simulink model "SMCControllerEH"  (R2022b)
settings: Solver=ode14x  StartTime=0.0  StopTime=simulationTime  FixedStep=sampleTime  RelTol=1e-6  AbsTol=1e-9
values from neighbouring files (symbols this model uses):
  chi = 0.05    [Basinofattraction.m]    (also in MainCEoptCase2_FOSMC.m; MainCEoptCase2_SMC.m; MainGAoptCase2_FOSMC.m; MainGAoptCase2_SMC.m)
  dxdisp0 = 0.0    (= 0)    [MainCEoptCase2_FOSMC.m]    (also in MainCEoptCase2_SMC.m; MainGAoptCase2_FOSMC.m; MainGAoptCase2_SMC.m)
  f_ref = 0.2    [Basinofattraction.m]    (also in MainCEoptCase2_FOSMC.m; MainCEoptCase2_SMC.m; MainGAoptCase2_FOSMC.m; MainGAoptCase2_SMC.m)
  fa = 0.2    [Basinofattraction.m]    (also in MainCEoptCase2_FOSMC.m; MainCEoptCase2_SMC.m; MainGAoptCase2_FOSMC.m; MainGAoptCase2_SMC.m)
  k = Xopt(1)    [Basinofattraction.m]    (also in MainCEoptCase2_FOSMC.m = x(1); MainCEoptCase2_SMC.m = x(1); MainGAoptCase2_FOSMC.m = x(1); MainGAoptCase2_SMC.m = x(1))
  kappa = 0.5    [Basinofattraction.m]    (also in MainCEoptCase2_FOSMC.m; MainCEoptCase2_SMC.m; MainGAoptCase2_FOSMC.m; MainGAoptCase2_SMC.m)
  ksi = 0.01    [Basinofattraction.m]    (also in MainCEoptCase2_FOSMC.m; MainCEoptCase2_SMC.m; MainGAoptCase2_FOSMC.m; MainGAoptCase2_SMC.m)
  lambda = 0.05    [Basinofattraction.m]    (also in MainCEoptCase2_FOSMC.m; MainCEoptCase2_SMC.m; MainGAoptCase2_FOSMC.m; MainGAoptCase2_SMC.m)
  lambda1 = Xopt(2)    [Basinofattraction.m]    (also in MainCEoptCase2_FOSMC.m = x(2); MainCEoptCase2_SMC.m = x(2); MainGAoptCase2_FOSMC.m = x(2); MainGAoptCase2_SMC.m = x(2))
  Omega_ref = 0.8    [Basinofattraction.m]    (also in MainCEoptCase2_FOSMC.m; MainCEoptCase2_SMC.m; MainGAoptCase2_FOSMC.m; MainGAoptCase2_SMC.m)
  sampleTime = 0.1    [Basinofattraction.m]    (also in MainCEoptCase2_FOSMC.m; MainCEoptCase2_SMC.m; MainGAoptCase2_FOSMC.m; MainGAoptCase2_SMC.m)
  xdisp0 = 1.0    (= 1)    [MainCEoptCase2_FOSMC.m]    (also in MainCEoptCase2_SMC.m; MainGAoptCase2_FOSMC.m; MainGAoptCase2_SMC.m)
settings Model: Creator=julio  LastModifiedBy=Usuario
settings SolverCC: AutoScaleAbsTol=off  InitialStep=sampleTime  AlgebraicLoopSolver=TrustRegion
settings DataIOCC: ReturnWorkspaceOutputs=off
settings OptimizationCC: LifeSpan=inf
settings DebuggingCC: UnconnectedInputMsg=warning  UnconnectedOutputMsg=warning  UnconnectedLineMsg=warning  SFUnexpectedBacktrackingDiag=warning  SFNoUnconditionalDefaultTransitionDiag=warning  SFMachineParentedDataDiag=warning  ArithmeticOperatorsInVariantConditions=warning
settings ModelReferenceCC: EnableRefExpFcnMdlSchedulingChecks=on
settings SFSimCC: SimUseLocalCustomCode=off  CustomCodeUndefinedFunction=UseInterfaceOnly
settings RTWCC: RTWUseLocalCustomCode=off
settings CodeAppCC: StateflowObjectComments=on
settings GRTTargetCC: TargetLangStandard=C89/C90 (ANSI)
settings ConfigComp: CovMetricSettings=dw  CovSaveCumulativeToWorkspaceVar=on  CovSaveSingleToWorkspaceVar=on  CovExternalEMLEnable=off

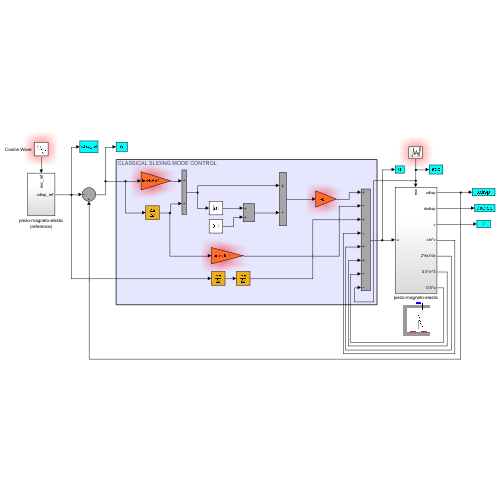
[thumbnail: Simulink's stored preview of the top-level diagram]
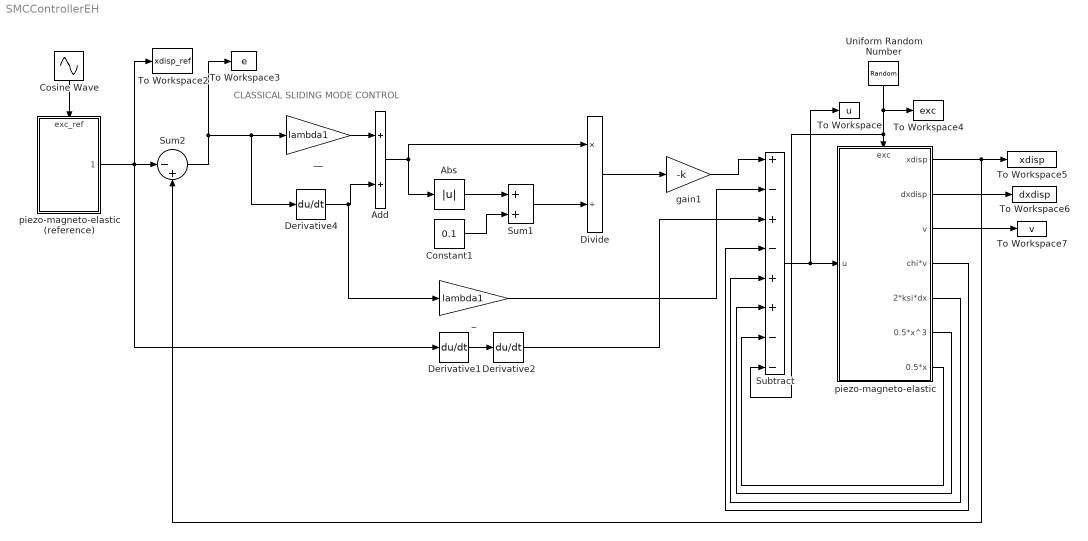
== system SMCControllerEH ==
  note: CLASSICAL SLIDING MODE CONTROL
  Abs : Abs  SaturateOnIntegerOverflow=off
  Add : Sum
  Constant1 : Constant  Value=0.1
  Cosine Wave : Sin  Amplitude=f_ref  Frequency=Omega_ref  SampleTime=0
  Derivative1 : Derivative
  Derivative2 : Derivative
  Derivative4 : Derivative
  Divide : Product  Inputs=*/
  Subtract : Sum  Inputs=+-+-++--
  Sum1 : Sum
  Sum2 : Sum  Inputs=|-+
  To Workspace : ToWorkspace  VariableName=u  SampleTime=-1
  To Workspace2 : ToWorkspace  VariableName=xdisp_ref  SampleTime=-1
  To Workspace3 : ToWorkspace  VariableName=e  SampleTime=-1
  To Workspace4 : ToWorkspace  VariableName=exc  SampleTime=-1
  To Workspace5 : ToWorkspace  VariableName=xdisp  SampleTime=-1
  To Workspace6 : ToWorkspace  VariableName=dxdisp  SampleTime=-1
  To Workspace7 : ToWorkspace  VariableName=v  SampleTime=-1
  Uniform Random Number : UniformRandomNumber  Minimum=-fa  Maximum=fa  Seed=1  SampleTime=sampleTime
  _ : Gain  Gain=lambda1
  __ : Gain  Gain=lambda1
  gain1 : Gain  Gain=-k
  piezo-magneto-elastic : Subsystem
      settings: PortSchema="{\"entries\":[{\"content\":{\"sides\":[{\"content\":{\"connectorIds\":[\"In1\"]},\"type\":\"ConnectorPlacement.EquallySpacedRectSide\",\"uuid\":\"c2ba6895-4fe1-43b2-9166-bfc98075714a\"},{\"content\":{\"connectorIds\":[\"Out1\",\"Out2\",\"Out3\",\"Out4\",\"Out5\",\"Out6\",\"Out7\"],\"side\":\"RIGHT\"},\"type\":\"ConnectorPlacement.EquallySpacedRectSide\",\"uuid\":\"f318010f-5345-4abb-8ec4-2c3ff83e3584\"},{\"content\":{\"connectorIds\":[\"In2\"],\"side\":\"TOP\"},\"type\":\"ConnectorPlacement.EquallySpacedRectSide\",\"uuid\":\"166745b2-692d-46bd-9a0d-c3d5b18ab8b7\"}]},\"type\":\"ConnectorPlacement.EquallySpacedConnector\",\"uuid\":\"a1a091f7-104a-4664-af8a-63d268c77923\"}],\"packageUris\":[\"http://schema.mathworks.com/mf0/Connector/R2020b\"],\"version\":\"1.0\"}"
  piezo-magneto-elastic (reference) : Subsystem
      settings: PortSchema="{\"entries\":[{\"content\":{\"sides\":[{\"content\":{\"connectorIds\":[]},\"type\":\"ConnectorPlacement.EquallySpacedRectSide\",\"uuid\":\"2fa27d44-66dd-459a-a915-b9e739ab4464\"},{\"content\":{\"connectorIds\":[\"Out1\"],\"side\":\"RIGHT\"},\"type\":\"ConnectorPlacement.EquallySpacedRectSide\",\"uuid\":\"143cbf88-99f3-4a4f-90c8-d8dcff3037ad\"},{\"content\":{\"connectorIds\":[\"In1\"],\"side\":\"TOP\"},\"type\":\"ConnectorPlacement.EquallySpacedRectSide\",\"uuid\":\"0f1da41b-b693-4442-9f27-75426a8f7a9a\"}]},\"type\":\"ConnectorPlacement.EquallySpacedConnector\",\"uuid\":\"82ec817d-257e-4c4b-88fa-5616da8b4759\"}],\"packageUris\":[\"http://schema.mathworks.com/mf0/Connector/R2020b\"],\"version\":\"1.0\"}"
  wires:
  Subtract/1 -> piezo-magneto-elastic/1(u), To Workspace/1
  __/1 -> Add/1
  Derivative4/1 -> _/1, Add/2
  gain1/1 -> Subtract/1
  Add/1 -> Divide/1, Abs/1
  Divide/1 -> gain1/1
  Abs/1 -> Sum1/1
  Sum1/1 -> Divide/2
  Constant1/1 -> Sum1/2
  Sum2/1 -> Derivative4/1, __/1, To Workspace3/1
  Derivative1/1 -> Derivative2/1
  Derivative2/1 -> Subtract/3
  _/1 -> Subtract/2
  piezo-magneto-elastic/4(chi*v) -> Subtract/4
  piezo-magneto-elastic/5(2*ksi*dx) -> Subtract/5
  piezo-magneto-elastic/6(0.5*x^3) -> Subtract/6
  piezo-magneto-elastic/7(0.5*x) -> Subtract/7
  piezo-magneto-elastic (reference)/1(xdisp_ref) -> To Workspace2/1, Sum2/1, Derivative1/1
  Cosine Wave/1 -> piezo-magneto-elastic (reference)/1(exc_ref)
  piezo-magneto-elastic/1(xdisp) -> Sum2/2, To Workspace5/1
  piezo-magneto-elastic/2(dxdisp) -> To Workspace6/1
  piezo-magneto-elastic/3(v) -> To Workspace7/1
  Uniform Random Number/1 -> Subtract/8, piezo-magneto-elastic/2(exc), To Workspace4/1

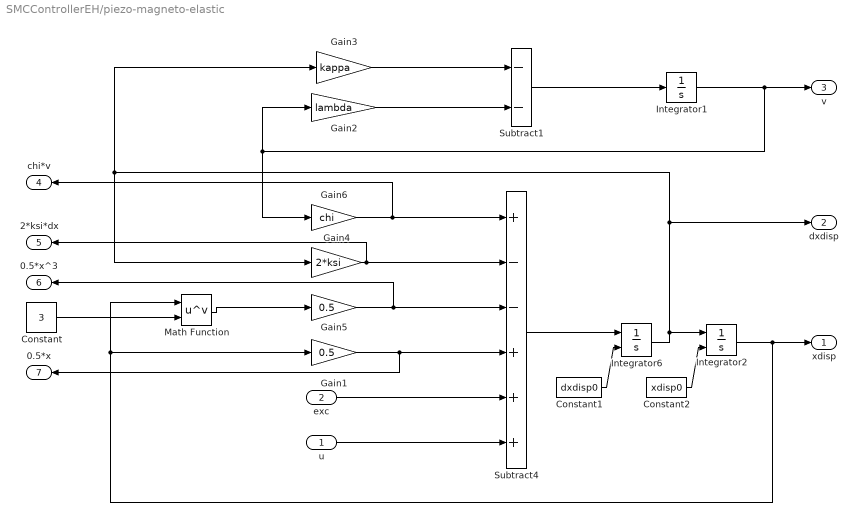
== system SMCControllerEH/piezo-magneto-elastic ==
  u : Inport
  exc : Inport  Port=2
  Constant : Constant  Value=3
  Constant1 : Constant  Value=dxdisp0
  Constant2 : Constant  Value=xdisp0
  Gain1 : Gain  Gain=0.5
  Gain2 : Gain  Gain=lambda
  Gain3 : Gain  Gain=kappa
  Gain4 : Gain  Gain=2*ksi
  Gain5 : Gain  Gain=0.5
  Gain6 : Gain  Gain=chi
  Integrator1 : Integrator
  Integrator2 : Integrator  InitialConditionSource=external  InitialCondition=1
  Integrator6 : Integrator  InitialConditionSource=external  InitialCondition=dxdisp0
  Math Function : Math  Operator=pow  SignedPower=on
  Subtract1 : Sum  Inputs=--
  Subtract4 : Sum  Inputs=+--+++
  xdisp : Outport
  dxdisp : Outport  Port=2
  v : Outport  Port=3
  chi*v : Outport  Port=4
  2*ksi*dx : Outport  Port=5
  0.5*x^3 : Outport  Port=6
  0.5*x : Outport  Port=7
  wires:
  Gain4/1 -> 2*ksi*dx/1, Subtract4/2
  Gain5/1 -> 0.5*x^3/1, Subtract4/3
  Math Function/1 -> Gain5/1
  Subtract4/1 -> Integrator6/1
  Gain1/1 -> 0.5*x/1, Subtract4/4
  Integrator6/1 -> dxdisp/1, Gain3/1, Gain4/1, Integrator2/1
  Subtract1/1 -> Integrator1/1
  Integrator1/1 -> v/1, Gain2/1, Gain6/1
  Gain2/1 -> Subtract1/2
  Gain6/1 -> Subtract4/1, chi*v/1
  Gain3/1 -> Subtract1/1
  Integrator2/1 -> xdisp/1, Math Function/1, Gain1/1
  Constant/1 -> Math Function/2
  u/1 -> Subtract4/6
  Constant1/1 -> Integrator6/2
  Constant2/1 -> Integrator2/2
  exc/1 -> Subtract4/5

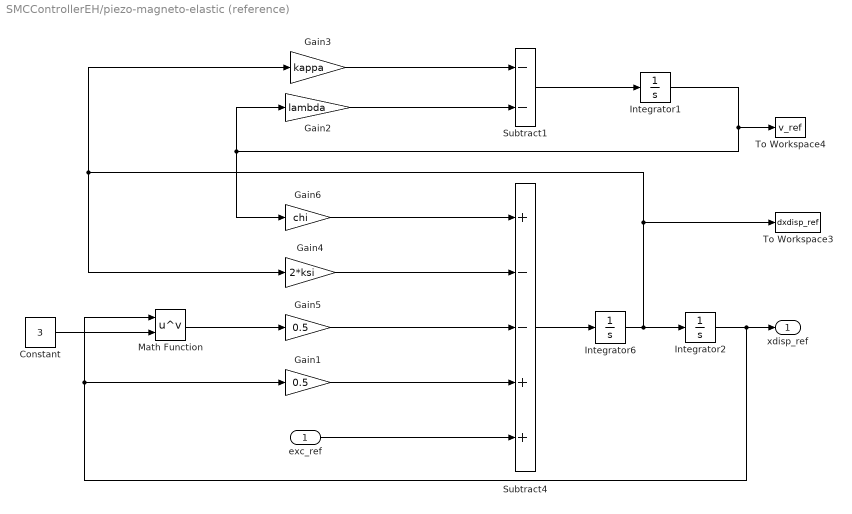
== system SMCControllerEH/piezo-magneto-elastic (reference) ==
  exc_ref : Inport
  Constant : Constant  Value=3
  Gain1 : Gain  Gain=0.5
  Gain2 : Gain  Gain=lambda
  Gain3 : Gain  Gain=kappa
  Gain4 : Gain  Gain=2*ksi
  Gain5 : Gain  Gain=0.5
  Gain6 : Gain  Gain=chi
  Integrator1 : Integrator
  Integrator2 : Integrator  InitialCondition=1
  Integrator6 : Integrator
  Math Function : Math  Operator=pow  SignedPower=on
  Subtract1 : Sum  Inputs=--
  Subtract4 : Sum  Inputs=+--++
  To Workspace3 : ToWorkspace  VariableName=dxdisp_ref  SampleTime=-1
  To Workspace4 : ToWorkspace  VariableName=v_ref  SampleTime=-1
  xdisp_ref : Outport
  wires:
  Gain4/1 -> Subtract4/2
  Gain5/1 -> Subtract4/3
  Math Function/1 -> Gain5/1
  Subtract4/1 -> Integrator6/1
  Gain1/1 -> Subtract4/4
  Integrator6/1 -> Integrator2/1, To Workspace3/1, Gain3/1, Gain4/1
  Subtract1/1 -> Integrator1/1
  Integrator1/1 -> Gain2/1, Gain6/1, To Workspace4/1
  Gain2/1 -> Subtract1/2
  Gain6/1 -> Subtract4/1
  Gain3/1 -> Subtract1/1
  Integrator2/1 -> Math Function/1, Gain1/1, xdisp_ref/1
  exc_ref/1 -> Subtract4/5
  Constant/1 -> Math Function/2
